simulink model "telemetry"  (R2026a)
settings: Solver=VariableStepAuto
libraries: simulink x1

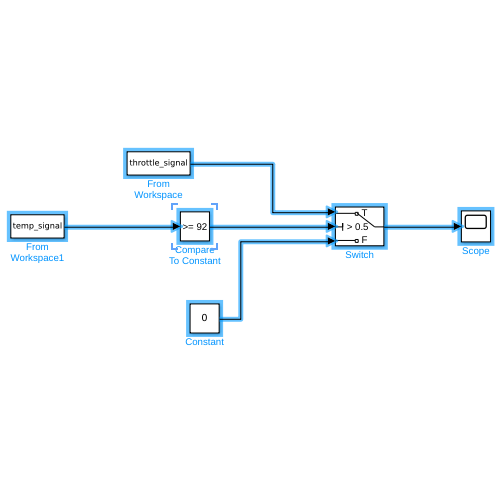
[thumbnail: Simulink's stored preview of the top-level diagram]
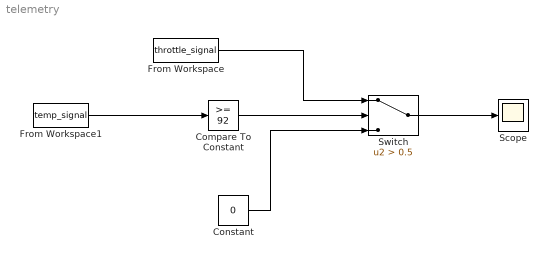
== system telemetry ==
  Compare To Constant : simulink/Logic and Bit Operations/Compare To Constant  relop=>=  const=92  OutDataTypeStr=boolean
  Constant : Constant  Value=0
  From Workspace : FromWorkspace  VariableName=throttle_signal
  From Workspace1 : FromWorkspace  VariableName=temp_signal
  Scope : Scope
      settings: ActiveDisplayYMinimum=-3.763749999999999  ActiveDisplayYMaximum=33.87375
  Switch : Switch  Criteria=u2 > Threshold  Threshold=0.5  SaturateOnIntegerOverflow=off  InputSameDT=off
  wires:
  From Workspace1/1 -> Compare To Constant/1
  Compare To Constant/1 -> Switch/2
  Constant/1 -> Switch/3
  From Workspace/1 -> Switch/1
  Switch/1 -> Scope/1
